simulink model "GS_model"  (R2018b)
settings: Solver=ode5  StartTime=0.0  StopTime=SimuStopTime  FixedStep=T_Simu  RelTol=1e-3
InitFcn:
  | Initial
undefined symbols (not defined in the file or in its folder): Aba10, Aba20, aeroCIP2006_S, aeroCIP2006_X, aeroCIP2006_Y, Agl0, Ass_kS, Ass_n1, Ass_n2, Ass_n3, Ass_n4, Ass_Noise, Ass_R, Ass_Resolution, Ass_TmOrder, AssA_Fix_Abs, AssB_Fix_Abs, AssC_Fix_Abs, AssD_Fix_Abs, AssE_Fix_Aps, AssF_Fix_Aps, C, c_max, c_min, Cd, CenterOfFigNX, CenterOfFigNY, CenterOfFigNZ, CenterOfFigP1, CenterOfFigP2, CenterOfFigPX, CenterOfFigPY, CenterOfFigPZ, Cmu, Crou, DEG2RAD, DiscIntNeverNeededParam, Eg_Dir, Eg_F, Eg_PrepareTime, Eg_r_L_L, Fw_Abf, Fw_Hmax, Fw_J, Fw_Spd0, Fw_Tmax, git_hash_BaseLine, git_hash_Project, Gnss_Noise_Pos, Gnss_Noise_Vel, Gnss_PropgationTime, GyroA_Fix_Abg, GyroA_Noise, GyroB_Fix_Abg, GyroB_Noise, GyroC_Fix_Abg, GyroC_Noise, GyroD_Fix_Abg, GyroD_Noise, h ... (+94)
libraries: simulink x308, sharedutil x46, aerolibutil x37, sharedtransform x31, vrlib x14, aerolibgravity2 x2
(part 18 of 20)

== system GS_model/Subsystem2/Subsystem/Sensor/Magnetometer/MmModel3/Mm_ErrSet/MmErrSet/MmErrSet_WildValue/MmAxisXErrSet_WildValue1 ==
  MmAxis_in : Inport
  ErrSwitch : Inport  Port=2
  MmAxis_Num : Inport  Port=3
  MmAxis_WildValue : Inport  Port=4
  Compare To Zero : simulink/Logic and Bit Operations/Compare To Zero  relop===  OutDataTypeStr=boolean
  Demux1 : Demux  Outputs=2
  Logical Operator : Logic  Operator=OR  AllPortsSameDT=off  OutDataTypeStr=boolean
  Relational Operator9 : RelationalOperator  Operator===  OutDataTypeStr=boolean  RndMeth=Simplest
  Switch1 : Switch  Criteria=u2 > Threshold  Threshold=0.5
  Triggered Subsystem8 : Subsystem  TreatAsAtomicUnit=on
  MmAxis_out : Outport
  wires:
  Logical Operator/1 -> Triggered Subsystem8/Enable
  Compare To Zero/1 -> Logical Operator/1
  Relational Operator9/1 -> Logical Operator/2
  Switch1/1 -> MmAxis_out/1
  MmAxis_in/1 -> Switch1/3
  Demux1/1 -> Relational Operator9/1, Compare To Zero/1
  Demux1/2 -> Triggered Subsystem8/1(In1)
  Triggered Subsystem8/1(Out1) -> Switch1/2
  MmAxis_Num/1 -> Relational Operator9/2
  MmAxis_WildValue/1 -> Switch1/1
  ErrSwitch/1 -> Demux1/1

== system GS_model/Subsystem2/Subsystem/Sensor/Magnetometer/MmModel3/Mm_ErrSet/MmErrSet/MmErrSet_WildValue/MmAxisXErrSet_WildValue2 ==
  MmAxis_in : Inport
  ErrSwitch : Inport  Port=2
  MmAxis_Num : Inport  Port=3
  MmAxis_WildValue : Inport  Port=4
  Compare To Zero : simulink/Logic and Bit Operations/Compare To Zero  relop===  OutDataTypeStr=boolean
  Demux1 : Demux  Outputs=2
  Logical Operator : Logic  Operator=OR  AllPortsSameDT=off  OutDataTypeStr=boolean
  Relational Operator9 : RelationalOperator  Operator===  OutDataTypeStr=boolean  RndMeth=Simplest
  Switch1 : Switch  Criteria=u2 > Threshold  Threshold=0.5
  Triggered Subsystem8 : Subsystem  TreatAsAtomicUnit=on
  MmAxis_out : Outport
  wires:
  ErrSwitch/1 -> Demux1/1
  MmAxis_WildValue/1 -> Switch1/1
  MmAxis_Num/1 -> Relational Operator9/2
  Triggered Subsystem8/1(Out1) -> Switch1/2
  Demux1/2 -> Triggered Subsystem8/1(In1)
  Demux1/1 -> Compare To Zero/1, Relational Operator9/1
  MmAxis_in/1 -> Switch1/3
  Switch1/1 -> MmAxis_out/1
  Relational Operator9/1 -> Logical Operator/2
  Compare To Zero/1 -> Logical Operator/1
  Logical Operator/1 -> Triggered Subsystem8/Enable

== system GS_model/Subsystem2/Subsystem/Sensor/Magnetometer/MmModel4/Mm_ErrSet/MmErrSet/MmErrSet_Constant/MmAxisXErrSet_Constant ==
  MmAxis_in : Inport
  ErrSwitch : Inport  Port=2
  MmAxis_Num : Inport  Port=3
  Compare To Zero : simulink/Logic and Bit Operations/Compare To Zero  relop===  OutDataTypeStr=boolean
  Demux1 : Demux  Outputs=2
  Logical Operator : Logic  Operator=OR  AllPortsSameDT=off  OutDataTypeStr=boolean
  Memory : Memory
  Relational Operator9 : RelationalOperator  Operator===  OutDataTypeStr=boolean  RndMeth=Simplest
  Switch1 : Switch  Criteria=u2 > Threshold  Threshold=0.5
  Triggered Subsystem8 : Subsystem  TreatAsAtomicUnit=on
  MmAxis_out : Outport
  wires:
  Logical Operator/1 -> Triggered Subsystem8/Enable
  Compare To Zero/1 -> Logical Operator/1
  Relational Operator9/1 -> Logical Operator/2
  MmAxis_Num/1 -> Relational Operator9/1
  Demux1/1 -> Relational Operator9/2, Compare To Zero/1
  Triggered Subsystem8/1(Out1) -> Switch1/2
  ErrSwitch/1 -> Demux1/1
  Memory/1 -> Switch1/1
  Demux1/2 -> Triggered Subsystem8/1(In1)
  MmAxis_in/1 -> Switch1/3
  Switch1/1 -> Memory/1, MmAxis_out/1

== system GS_model/Subsystem2/Subsystem/Sensor/Magnetometer/MmModel4/Mm_ErrSet/MmErrSet/MmErrSet_Constant/MmAxisXErrSet_Constant1 ==
  MmAxis_in : Inport
  ErrSwitch : Inport  Port=2
  MmAxis_Num : Inport  Port=3
  Compare To Zero : simulink/Logic and Bit Operations/Compare To Zero  relop===  OutDataTypeStr=boolean
  Demux1 : Demux  Outputs=2
  Logical Operator : Logic  Operator=OR  AllPortsSameDT=off  OutDataTypeStr=boolean
  Memory : Memory
  Relational Operator9 : RelationalOperator  Operator===  OutDataTypeStr=boolean  RndMeth=Simplest
  Switch1 : Switch  Criteria=u2 > Threshold  Threshold=0.5
  Triggered Subsystem8 : Subsystem  TreatAsAtomicUnit=on
  MmAxis_out : Outport
  wires:
  Switch1/1 -> MmAxis_out/1, Memory/1
  MmAxis_in/1 -> Switch1/3
  Demux1/2 -> Triggered Subsystem8/1(In1)
  Memory/1 -> Switch1/1
  ErrSwitch/1 -> Demux1/1
  Triggered Subsystem8/1(Out1) -> Switch1/2
  Demux1/1 -> Compare To Zero/1, Relational Operator9/2
  MmAxis_Num/1 -> Relational Operator9/1
  Relational Operator9/1 -> Logical Operator/2
  Compare To Zero/1 -> Logical Operator/1
  Logical Operator/1 -> Triggered Subsystem8/Enable

== system GS_model/Subsystem2/Subsystem/Sensor/Magnetometer/MmModel4/Mm_ErrSet/MmErrSet/MmErrSet_Constant/MmAxisXErrSet_Constant2 ==
  MmAxis_in : Inport
  ErrSwitch : Inport  Port=2
  MmAxis_Num : Inport  Port=3
  Compare To Zero : simulink/Logic and Bit Operations/Compare To Zero  relop===  OutDataTypeStr=boolean
  Demux1 : Demux  Outputs=2
  Logical Operator : Logic  Operator=OR  AllPortsSameDT=off  OutDataTypeStr=boolean
  Memory : Memory
  Relational Operator9 : RelationalOperator  Operator===  OutDataTypeStr=boolean  RndMeth=Simplest
  Switch1 : Switch  Criteria=u2 > Threshold  Threshold=0.5
  Triggered Subsystem8 : Subsystem  TreatAsAtomicUnit=on
  MmAxis_out : Outport
  wires:
  Logical Operator/1 -> Triggered Subsystem8/Enable
  Compare To Zero/1 -> Logical Operator/1
  Relational Operator9/1 -> Logical Operator/2
  MmAxis_Num/1 -> Relational Operator9/1
  Demux1/1 -> Relational Operator9/2, Compare To Zero/1
  Triggered Subsystem8/1(Out1) -> Switch1/2
  ErrSwitch/1 -> Demux1/1
  Memory/1 -> Switch1/1
  Demux1/2 -> Triggered Subsystem8/1(In1)
  MmAxis_in/1 -> Switch1/3
  Switch1/1 -> Memory/1, MmAxis_out/1

== system GS_model/Subsystem2/Subsystem/Sensor/Magnetometer/MmModel4/Mm_ErrSet/MmErrSet/MmErrSet_Jump/MmAxisXErrSet_Jump ==
  MmAxis_in : Inport
  ErrSet : Inport  Port=2
  MmAxis_Num : Inport  Port=3
  MmAxis_JumpSet : Inport  Port=4
  Add : Sum  Inputs=|++
  Compare To Zero : simulink/Logic and Bit Operations/Compare To Zero  relop===  OutDataTypeStr=boolean
  Demux1 : Demux
  Logical Operator : Logic  Operator=OR  AllPortsSameDT=off  OutDataTypeStr=boolean
  Product : Product
  Relational Operator9 : RelationalOperator  Operator===  OutDataTypeStr=boolean  RndMeth=Simplest
  Switch3 : Switch  Criteria=u2 > Threshold  Threshold=0.5
  Terminator : Terminator
  Triggered Subsystem8 : Subsystem  TreatAsAtomicUnit=on
  MmAxis_out : Outport
  wires:
  Logical Operator/1 -> Triggered Subsystem8/Enable
  Compare To Zero/1 -> Logical Operator/1
  Relational Operator9/1 -> Logical Operator/2
  Demux1/1 -> Relational Operator9/1, Compare To Zero/1  "Axis"
  Demux1/4 -> Product/2  "Coff"
  Triggered Subsystem8/1(Out1) -> Switch3/2
  Product/1 -> Add/1
  Demux1/2 -> Triggered Subsystem8/1(In1)  "Switch"
  MmAxis_in/1 -> Switch3/3, Add/2
  ErrSet/1 -> Demux1/1
  Add/1 -> Switch3/1
  Demux1/3 -> Terminator/1  "Period"
  MmAxis_Num/1 -> Relational Operator9/2
  Switch3/1 -> MmAxis_out/1
  MmAxis_JumpSet/1 -> Product/1

== system GS_model/Subsystem2/Subsystem/Sensor/Magnetometer/MmModel4/Mm_ErrSet/MmErrSet/MmErrSet_Jump/MmAxisXErrSet_Jump1 ==
  MmAxis_in : Inport
  ErrSet : Inport  Port=2
  MmAxis_Num : Inport  Port=3
  MmAxis_JumpSet : Inport  Port=4
  Add : Sum  Inputs=|++
  Compare To Zero : simulink/Logic and Bit Operations/Compare To Zero  relop===  OutDataTypeStr=boolean
  Demux1 : Demux
  Logical Operator : Logic  Operator=OR  AllPortsSameDT=off  OutDataTypeStr=boolean
  Product : Product
  Relational Operator9 : RelationalOperator  Operator===  OutDataTypeStr=boolean  RndMeth=Simplest
  Switch3 : Switch  Criteria=u2 > Threshold  Threshold=0.5
  Terminator : Terminator
  Triggered Subsystem8 : Subsystem  TreatAsAtomicUnit=on
  MmAxis_out : Outport
  wires:
  MmAxis_JumpSet/1 -> Product/1
  Switch3/1 -> MmAxis_out/1
  MmAxis_Num/1 -> Relational Operator9/2
  Demux1/3 -> Terminator/1  "Period"
  Add/1 -> Switch3/1
  ErrSet/1 -> Demux1/1
  MmAxis_in/1 -> Add/2, Switch3/3
  Demux1/2 -> Triggered Subsystem8/1(In1)  "Switch"
  Product/1 -> Add/1
  Triggered Subsystem8/1(Out1) -> Switch3/2
  Demux1/4 -> Product/2  "Coff"
  Demux1/1 -> Compare To Zero/1, Relational Operator9/1  "Axis"
  Relational Operator9/1 -> Logical Operator/2
  Compare To Zero/1 -> Logical Operator/1
  Logical Operator/1 -> Triggered Subsystem8/Enable

== system GS_model/Subsystem2/Subsystem/Sensor/Magnetometer/MmModel4/Mm_ErrSet/MmErrSet/MmErrSet_Jump/MmAxisXErrSet_Jump2 ==
  MmAxis_in : Inport
  ErrSet : Inport  Port=2
  MmAxis_Num : Inport  Port=3
  MmAxis_JumpSet : Inport  Port=4
  Add : Sum  Inputs=|++
  Compare To Zero : simulink/Logic and Bit Operations/Compare To Zero  relop===  OutDataTypeStr=boolean
  Demux1 : Demux
  Logical Operator : Logic  Operator=OR  AllPortsSameDT=off  OutDataTypeStr=boolean
  Product : Product
  Relational Operator9 : RelationalOperator  Operator===  OutDataTypeStr=boolean  RndMeth=Simplest
  Switch3 : Switch  Criteria=u2 > Threshold  Threshold=0.5
  Terminator : Terminator
  Triggered Subsystem8 : Subsystem  TreatAsAtomicUnit=on
  MmAxis_out : Outport
  wires:
  Logical Operator/1 -> Triggered Subsystem8/Enable
  Compare To Zero/1 -> Logical Operator/1
  Relational Operator9/1 -> Logical Operator/2
  Demux1/1 -> Relational Operator9/1, Compare To Zero/1  "Axis"
  Demux1/4 -> Product/2  "Coff"
  Triggered Subsystem8/1(Out1) -> Switch3/2
  Product/1 -> Add/1
  Demux1/2 -> Triggered Subsystem8/1(In1)  "Switch"
  MmAxis_in/1 -> Switch3/3, Add/2
  ErrSet/1 -> Demux1/1
  Add/1 -> Switch3/1
  Demux1/3 -> Terminator/1  "Period"
  MmAxis_Num/1 -> Relational Operator9/2
  Switch3/1 -> MmAxis_out/1
  MmAxis_JumpSet/1 -> Product/1

== system GS_model/Subsystem2/Subsystem/Sensor/Magnetometer/MmModel4/Mm_ErrSet/MmErrSet/MmErrSet_Wave/MmAxisXErrSet_Wave ==
  MmAxis_in : Inport
  ErrSet : Inport  Port=2
  MmAxis_Num : Inport  Port=3
  MmAxis_WaveSet : Inport  Port=4
  Add : Sum  Inputs=|++
  Compare To Zero : simulink/Logic and Bit Operations/Compare To Zero  relop===  OutDataTypeStr=boolean
  Demux1 : Demux  Outputs=3
  Logical Operator : Logic  Operator=OR  AllPortsSameDT=off  OutDataTypeStr=boolean
  Product : Product
  Relational Operator9 : RelationalOperator  Operator===  OutDataTypeStr=boolean  RndMeth=Simplest
  Switch3 : Switch  Criteria=u2 > Threshold  Threshold=0.5
  Triggered Subsystem8 : Subsystem  TreatAsAtomicUnit=on
  MmAxis_out : Outport
  wires:
  Compare To Zero/1 -> Logical Operator/1
  Logical Operator/1 -> Triggered Subsystem8/Enable
  Relational Operator9/1 -> Logical Operator/2
  MmAxis_WaveSet/1 -> Product/1
  Product/1 -> Add/1
  ErrSet/1 -> Demux1/1
  Add/1 -> Switch3/1
  MmAxis_in/1 -> Add/2, Switch3/3
  Demux1/2 -> Triggered Subsystem8/1(In1)  "Switch"
  Demux1/1 -> Relational Operator9/1, Compare To Zero/1  "Axis"
  Demux1/3 -> Product/2  "Coff"
  MmAxis_Num/1 -> Relational Operator9/2
  Switch3/1 -> MmAxis_out/1
  Triggered Subsystem8/1(Out1) -> Switch3/2

== system GS_model/Subsystem2/Subsystem/Sensor/Magnetometer/MmModel4/Mm_ErrSet/MmErrSet/MmErrSet_Wave/MmAxisXErrSet_Wave1 ==
  MmAxis_in : Inport
  ErrSet : Inport  Port=2
  MmAxis_Num : Inport  Port=3
  MmAxis_WaveSet : Inport  Port=4
  Add : Sum  Inputs=|++
  Compare To Zero : simulink/Logic and Bit Operations/Compare To Zero  relop===  OutDataTypeStr=boolean
  Demux1 : Demux  Outputs=3
  Logical Operator : Logic  Operator=OR  AllPortsSameDT=off  OutDataTypeStr=boolean
  Product : Product
  Relational Operator9 : RelationalOperator  Operator===  OutDataTypeStr=boolean  RndMeth=Simplest
  Switch3 : Switch  Criteria=u2 > Threshold  Threshold=0.5
  Triggered Subsystem8 : Subsystem  TreatAsAtomicUnit=on
  MmAxis_out : Outport
  wires:
  Triggered Subsystem8/1(Out1) -> Switch3/2
  Switch3/1 -> MmAxis_out/1
  MmAxis_Num/1 -> Relational Operator9/2
  Demux1/3 -> Product/2  "Coff"
  Demux1/1 -> Compare To Zero/1, Relational Operator9/1  "Axis"
  Demux1/2 -> Triggered Subsystem8/1(In1)  "Switch"
  MmAxis_in/1 -> Switch3/3, Add/2
  Add/1 -> Switch3/1
  ErrSet/1 -> Demux1/1
  Product/1 -> Add/1
  MmAxis_WaveSet/1 -> Product/1
  Relational Operator9/1 -> Logical Operator/2
  Logical Operator/1 -> Triggered Subsystem8/Enable
  Compare To Zero/1 -> Logical Operator/1

== system GS_model/Subsystem2/Subsystem/Sensor/Magnetometer/MmModel4/Mm_ErrSet/MmErrSet/MmErrSet_Wave/MmAxisXErrSet_Wave2 ==
  MmAxis_in : Inport
  ErrSet : Inport  Port=2
  MmAxis_Num : Inport  Port=3
  MmAxis_WaveSet : Inport  Port=4
  Add : Sum  Inputs=|++
  Compare To Zero : simulink/Logic and Bit Operations/Compare To Zero  relop===  OutDataTypeStr=boolean
  Demux1 : Demux  Outputs=3
  Logical Operator : Logic  Operator=OR  AllPortsSameDT=off  OutDataTypeStr=boolean
  Product : Product
  Relational Operator9 : RelationalOperator  Operator===  OutDataTypeStr=boolean  RndMeth=Simplest
  Switch3 : Switch  Criteria=u2 > Threshold  Threshold=0.5
  Triggered Subsystem8 : Subsystem  TreatAsAtomicUnit=on
  MmAxis_out : Outport
  wires:
  Compare To Zero/1 -> Logical Operator/1
  Logical Operator/1 -> Triggered Subsystem8/Enable
  Relational Operator9/1 -> Logical Operator/2
  MmAxis_WaveSet/1 -> Product/1
  Product/1 -> Add/1
  ErrSet/1 -> Demux1/1
  Add/1 -> Switch3/1
  MmAxis_in/1 -> Add/2, Switch3/3
  Demux1/2 -> Triggered Subsystem8/1(In1)  "Switch"
  Demux1/1 -> Relational Operator9/1, Compare To Zero/1  "Axis"
  Demux1/3 -> Product/2  "Coff"
  MmAxis_Num/1 -> Relational Operator9/2
  Switch3/1 -> MmAxis_out/1
  Triggered Subsystem8/1(Out1) -> Switch3/2

== system GS_model/Subsystem2/Subsystem/Sensor/Magnetometer/MmModel4/Mm_ErrSet/MmErrSet/MmErrSet_WildValue/MmAxisXErrSet_WildValue ==
  MmAxis_in : Inport
  ErrSwitch : Inport  Port=2
  MmAxis_Num : Inport  Port=3
  MmAxis_WildValue : Inport  Port=4
  Compare To Zero : simulink/Logic and Bit Operations/Compare To Zero  relop===  OutDataTypeStr=boolean
  Demux1 : Demux  Outputs=2
  Logical Operator : Logic  Operator=OR  AllPortsSameDT=off  OutDataTypeStr=boolean
  Relational Operator9 : RelationalOperator  Operator===  OutDataTypeStr=boolean  RndMeth=Simplest
  Switch1 : Switch  Criteria=u2 > Threshold  Threshold=0.5
  Triggered Subsystem8 : Subsystem  TreatAsAtomicUnit=on
  MmAxis_out : Outport
  wires:
  Logical Operator/1 -> Triggered Subsystem8/Enable
  Compare To Zero/1 -> Logical Operator/1
  Relational Operator9/1 -> Logical Operator/2
  Switch1/1 -> MmAxis_out/1
  MmAxis_in/1 -> Switch1/3
  Demux1/1 -> Relational Operator9/1, Compare To Zero/1
  Demux1/2 -> Triggered Subsystem8/1(In1)
  Triggered Subsystem8/1(Out1) -> Switch1/2
  MmAxis_Num/1 -> Relational Operator9/2
  MmAxis_WildValue/1 -> Switch1/1
  ErrSwitch/1 -> Demux1/1

== system GS_model/Subsystem2/Subsystem/Sensor/Magnetometer/MmModel4/Mm_ErrSet/MmErrSet/MmErrSet_WildValue/MmAxisXErrSet_WildValue1 ==
  MmAxis_in : Inport
  ErrSwitch : Inport  Port=2
  MmAxis_Num : Inport  Port=3
  MmAxis_WildValue : Inport  Port=4
  Compare To Zero : simulink/Logic and Bit Operations/Compare To Zero  relop===  OutDataTypeStr=boolean
  Demux1 : Demux  Outputs=2
  Logical Operator : Logic  Operator=OR  AllPortsSameDT=off  OutDataTypeStr=boolean
  Relational Operator9 : RelationalOperator  Operator===  OutDataTypeStr=boolean  RndMeth=Simplest
  Switch1 : Switch  Criteria=u2 > Threshold  Threshold=0.5
  Triggered Subsystem8 : Subsystem  TreatAsAtomicUnit=on
  MmAxis_out : Outport
  wires:
  ErrSwitch/1 -> Demux1/1
  MmAxis_WildValue/1 -> Switch1/1
  MmAxis_Num/1 -> Relational Operator9/2
  Triggered Subsystem8/1(Out1) -> Switch1/2
  Demux1/2 -> Triggered Subsystem8/1(In1)
  Demux1/1 -> Compare To Zero/1, Relational Operator9/1
  MmAxis_in/1 -> Switch1/3
  Switch1/1 -> MmAxis_out/1
  Relational Operator9/1 -> Logical Operator/2
  Compare To Zero/1 -> Logical Operator/1
  Logical Operator/1 -> Triggered Subsystem8/Enable

== system GS_model/Subsystem2/Subsystem/Sensor/Magnetometer/MmModel4/Mm_ErrSet/MmErrSet/MmErrSet_WildValue/MmAxisXErrSet_WildValue2 ==
  MmAxis_in : Inport
  ErrSwitch : Inport  Port=2
  MmAxis_Num : Inport  Port=3
  MmAxis_WildValue : Inport  Port=4
  Compare To Zero : simulink/Logic and Bit Operations/Compare To Zero  relop===  OutDataTypeStr=boolean
  Demux1 : Demux  Outputs=2
  Logical Operator : Logic  Operator=OR  AllPortsSameDT=off  OutDataTypeStr=boolean
  Relational Operator9 : RelationalOperator  Operator===  OutDataTypeStr=boolean  RndMeth=Simplest
  Switch1 : Switch  Criteria=u2 > Threshold  Threshold=0.5
  Triggered Subsystem8 : Subsystem  TreatAsAtomicUnit=on
  MmAxis_out : Outport
  wires:
  Logical Operator/1 -> Triggered Subsystem8/Enable
  Compare To Zero/1 -> Logical Operator/1
  Relational Operator9/1 -> Logical Operator/2
  Switch1/1 -> MmAxis_out/1
  MmAxis_in/1 -> Switch1/3
  Demux1/1 -> Relational Operator9/1, Compare To Zero/1
  Demux1/2 -> Triggered Subsystem8/1(In1)
  Triggered Subsystem8/1(Out1) -> Switch1/2
  MmAxis_Num/1 -> Relational Operator9/2
  MmAxis_WildValue/1 -> Switch1/1
  ErrSwitch/1 -> Demux1/1

== system GS_model/Subsystem2/Subsystem/PhysicsModel/Environment/Sun  press torque/Sun  press torque2/Sun  press torque/+Y SunPanel/Compute press of sun radiation/1//r ==
  In1 : Inport
  If : If  IfExpression=u1== 0
  If Action Subsystem1 : Subsystem  TreatAsAtomicUnit=on
  If Action Subsystem2 : Subsystem  TreatAsAtomicUnit=on
  Merge : Merge
  Out1 : Outport
  wires:
  In1/1 -> If Action Subsystem1/1(In1), If/1
  Merge/1 -> Out1/1
  If Action Subsystem2/1(Out1) -> Merge/1
  If Action Subsystem1/1(Out1) -> Merge/2
  If/2 -> If Action Subsystem1/Action
  If/1 -> If Action Subsystem2/Action

== system GS_model/Subsystem2/Subsystem/PhysicsModel/Environment/Sun  press torque/Sun  press torque2/Sun  press torque/-Y SunPanel/Compute press of sun radiation/1//r ==
  In1 : Inport
  If : If  IfExpression=u1== 0
  If Action Subsystem1 : Subsystem  TreatAsAtomicUnit=on
  If Action Subsystem2 : Subsystem  TreatAsAtomicUnit=on
  Merge : Merge
  Out1 : Outport
  wires:
  If/1 -> If Action Subsystem2/Action
  If/2 -> If Action Subsystem1/Action
  If Action Subsystem1/1(Out1) -> Merge/2
  If Action Subsystem2/1(Out1) -> Merge/1
  Merge/1 -> Out1/1
  In1/1 -> If/1, If Action Subsystem1/1(In1)

== system GS_model/Subsystem2/Subsystem/PhysicsModel/Environment/Sun  press torque/Sun  press torque2/Sun  press torque/Torque from   satalite board/Torque from  board perpendicular to z axis /Compute press of sun radiation ==
  note: u_n
  note: u_t
  Sun Orientation : Inport
  TC_SunPressCoeff : Inport  Port=2
  1/r : Subsystem  TreatAsAtomicUnit=on
  3x3 Cross Product : sharedutil/3x3 Cross Product  aMode=aMode
      settings: SourceProductBaseCode=AE,PW,MT,VE,VP
  3x3 Cross Product1 : sharedutil/3x3 Cross Product  aMode=aMode
      settings: SourceProductBaseCode=AE,PW,MT,VE,VP
  Board Orientation : Constant  Value=n_NZ  VectorParams1D=off
  Board Orientation1 : Constant  Value=n_PZ  VectorParams1D=off
  Board Orientation2 : Constant  Value=Szp_board  VectorParams1D=off
  Board Orientation3 : Constant  Value=Szn_board  VectorParams1D=off
  Crd2 : Constant  Value=2/3*Crou*Cmu
  Dot Product : DotProduct  InputSameDT=on  OutDataTypeStr=Inherit: Inherit via internal rule
  Dot Product1 : DotProduct  InputSameDT=on  OutDataTypeStr=Inherit: Inherit via internal rule
  Fcn : Fcn  Expr=u(3)
  Fcn1 : Fcn  Expr=u(3)
  Gain : Gain  Gain=1+Crou*(1-Cmu)
  Gain1 : Gain  Gain=-1  SaturateOnIntegerOverflow=on  OutDataTypeStr=Inherit: Same as input  ParamDataTypeStr=Inherit: Same as input
  Gain2 : Gain  Gain=SConst/C
  Gain3 : Gain  Gain=1-Crou+Crou*Cmu
  Product{1..6} (6 alike) : Product  SaturateOnIntegerOverflow=on  OutDataTypeStr=Inherit: Same as first input
  Sum1 : Sum  SaturateOnIntegerOverflow=on  InputSameDT=on  OutDataTypeStr=Inherit: Same as first input
  Sum2 : Sum  Inputs=|++  SaturateOnIntegerOverflow=on  InputSameDT=on  OutDataTypeStr=Inherit: Same as first input
  Switch1 : Switch  SaturateOnIntegerOverflow=on  InputSameDT=on
  Switch2 : Switch  SaturateOnIntegerOverflow=on  InputSameDT=on
  Trigonometric Function1 : Trigonometry
  Trigonometric Function2 : Trigonometry  Operator=acos
  Fz : Outport
  wires:
  Board Orientation1/1 -> Switch2/1
  Board Orientation/1 -> Switch2/3
  Fcn/1 -> Switch2/2
  Gain/1 -> Sum2/1
  Sum2/1 -> Product4/1
  Crd2/1 -> Sum2/2
  Gain1/1 -> Product4/2
  Switch2/1 -> Dot Product/2, Gain1/1, 3x3 Cross Product1/2, 3x3 Cross Product/2
  Sum1/1 -> Product3/1
  Sun Orientation/1 -> Fcn1/1, Fcn/1, 3x3 Cross Product/1, Dot Product/1
  Trigonometric Function2/1 -> Trigonometric Function1/1
  Gain3/1 -> Product2/2
  3x3 Cross Product/1 -> 3x3 Cross Product1/1
  1/r/1(Out1) -> Product1/2
  3x3 Cross Product1/1 -> Dot Product1/1, Product1/1, Dot Product1/2
  Product2/1 -> Sum1/1
  Product4/1 -> Sum1/2
  Product1/1 -> Product2/1
  Trigonometric Function1/1 -> Gain3/1
  Dot Product1/1 -> 1/r/1(In1)
  Product3/1 -> Fz/1
  Board Orientation2/1 -> Switch1/1
  Board Orientation3/1 -> Switch1/3
  Fcn1/1 -> Switch1/2
  Dot Product/1 -> Product5/2, Gain/1, Trigonometric Function2/1
  Product5/1 -> Gain2/1
  Switch1/1 -> Product5/1
  Gain2/1 -> Product6/1
  TC_SunPressCoeff/1 -> Product6/2
  Product6/1 -> Product3/2

== system GS_model/Subsystem2/Subsystem/PhysicsModel/Environment/Sun  press torque/Sun  press torque2/Sun  press torque/Torque from   satalite board/Torque from  board perpendicular to z axis /compute centroi 1 ==
  Orientation : Inport
  Cent : Inport  Port=2
  Fcn : Fcn  Expr=u(3)
  Sum2 : Sum  Inputs=|+-
  Switch1 : Switch  SaturateOnIntegerOverflow=on  InputSameDT=on
  y2 : Constant  Value=CenterOfFigNZ  VectorParams1D=off
  y3 : Constant  Value=CenterOfFigPZ  VectorParams1D=off
  r_z : Outport
  wires:
  Sum2/1 -> r_z/1
  y3/1 -> Switch1/1
  y2/1 -> Switch1/3
  Fcn/1 -> Switch1/2
  Orientation/1 -> Fcn/1
  Cent/1 -> Sum2/2
  Switch1/1 -> Sum2/1

== system GS_model/Subsystem2/Subsystem/PhysicsModel/Environment/Sun  press torque/Sun  press torque2/Sun  press torque/Torque from   satalite board/Torque from board perpendicular to x axis/Compute press of sun radiation ==
  note: cos_theta
  note: u_n
  note: u_t
  note: Huang zhen gui P67
  Sun Orientation : Inport
  TC_SunPressCoeff : Inport  Port=2
  1/r : Subsystem  TreatAsAtomicUnit=on
  3x3 Cross Product : sharedutil/3x3 Cross Product  aMode=aMode
      settings: SourceProductBaseCode=AE,PW,MT,VE,VP
  3x3 Cross Product1 : sharedutil/3x3 Cross Product  aMode=aMode
      settings: SourceProductBaseCode=AE,PW,MT,VE,VP
  Board Orientation : Constant  Value=n_NX  VectorParams1D=off
  Board Orientation1 : Constant  Value=n_PX  VectorParams1D=off
  Crd2 : Constant  Value=2/3*Crou*Cmu
  Dot Product : DotProduct  InputSameDT=on  OutDataTypeStr=Inherit: Inherit via internal rule
  Dot Product1 : DotProduct  InputSameDT=on  OutDataTypeStr=Inherit: Inherit via internal rule
  Fcn : Fcn  Expr=u(1)
  Gain : Gain  Gain=1+Crou*(1-Cmu)
  Gain1 : Gain  Gain=-1  SaturateOnIntegerOverflow=on  OutDataTypeStr=Inherit: Same as input  ParamDataTypeStr=Inherit: Same as input
  Gain2 : Gain  Gain=SConst/C*Sx_board
  Gain4 : Gain  Gain=1-Crou+Crou*Cmu
  Product : Product
  Product{1..4} (4 alike) : Product  SaturateOnIntegerOverflow=on  OutDataTypeStr=Inherit: Same as first input
  Sum1 : Sum  SaturateOnIntegerOverflow=on  InputSameDT=on  OutDataTypeStr=Inherit: Same as first input
  Sum2 : Sum  Inputs=|++  SaturateOnIntegerOverflow=on  InputSameDT=on  OutDataTypeStr=Inherit: Same as first input
  Switch2 : Switch  SaturateOnIntegerOverflow=on  InputSameDT=on
  Trigonometric Function1 : Trigonometry
  Trigonometric Function2 : Trigonometry  Operator=acos
  Fx : Outport
  wires:
  Board Orientation1/1 -> Switch2/1
  Board Orientation/1 -> Switch2/3
  Fcn/1 -> Switch2/2
  Gain/1 -> Sum2/1
  Sum2/1 -> Product4/1
  Crd2/1 -> Sum2/2
  Gain1/1 -> Product4/2
  Switch2/1 -> Gain1/1, 3x3 Cross Product1/2, 3x3 Cross Product/2, Dot Product/1
  Sum1/1 -> Product3/1
  Dot Product/1 -> Gain2/1, Gain/1, Trigonometric Function2/1
  Sun Orientation/1 -> Fcn/1, Dot Product/2, 3x3 Cross Product/1
  Trigonometric Function2/1 -> Trigonometric Function1/1
  Gain4/1 -> Product2/2
  3x3 Cross Product/1 -> 3x3 Cross Product1/1
  1/r/1(Out1) -> Product1/2
  3x3 Cross Product1/1 -> Dot Product1/2, Dot Product1/1, Product1/1
  Product3/1 -> Fx/1
  Product2/1 -> Sum1/1
  Product4/1 -> Sum1/2
  Product1/1 -> Product2/1
  Trigonometric Function1/1 -> Gain4/1
  Dot Product1/1 -> 1/r/1(In1)
  Gain2/1 -> Product/1
  TC_SunPressCoeff/1 -> Product/2
  Product/1 -> Product3/2

== system GS_model/Subsystem2/Subsystem/PhysicsModel/Environment/Sun  press torque/Sun  press torque2/Sun  press torque/Torque from   satalite board/Torque from board perpendicular to x axis/compute centroi 1 ==
  Orientation : Inport
  Cent : Inport  Port=2
  Fcn : Fcn  Expr=u(1)
  Sum2 : Sum  Inputs=|+-
  Switch1 : Switch  SaturateOnIntegerOverflow=on  InputSameDT=on
  y2 : Constant  Value=CenterOfFigNX  VectorParams1D=off
  y3 : Constant  Value=CenterOfFigPX  VectorParams1D=off
  r_x : Outport
  wires:
  Sum2/1 -> r_x/1
  y3/1 -> Switch1/1
  y2/1 -> Switch1/3
  Fcn/1 -> Switch1/2
  Orientation/1 -> Fcn/1
  Cent/1 -> Sum2/2
  Switch1/1 -> Sum2/1

== system GS_model/Subsystem2/Subsystem/PhysicsModel/Environment/Sun  press torque/Sun  press torque2/Sun  press torque/Torque from   satalite board/Torque from board perpendicular to y axis/Compute press of sun radiation1 ==
  note: cos_theta
  note: u_n
  note: u_t
  note: Huang zhen gui P67
  Sun Orientation : Inport
  TC_SunPressCoeff : Inport  Port=2
  1/r : Subsystem  TreatAsAtomicUnit=on
  3x3 Cross Product : sharedutil/3x3 Cross Product  aMode=aMode
      settings: SourceProductBaseCode=AE,PW,MT,VE,VP
  3x3 Cross Product1 : sharedutil/3x3 Cross Product  aMode=aMode
      settings: SourceProductBaseCode=AE,PW,MT,VE,VP
  Board Orientation : Constant  Value=n_NY  VectorParams1D=off
  Board Orientation1 : Constant  Value=n_PY  VectorParams1D=off
  Crd2 : Constant  Value=2/3*Crou*Cmu
  Dot Product : DotProduct  InputSameDT=on  OutDataTypeStr=Inherit: Inherit via internal rule
  Dot Product1 : DotProduct  InputSameDT=on  OutDataTypeStr=Inherit: Inherit via internal rule
  Fcn : Fcn  Expr=u(2)
  Gain : Gain  Gain=1+Crou*(1-Cmu)
  Gain1 : Gain  Gain=-1  SaturateOnIntegerOverflow=on  OutDataTypeStr=Inherit: Same as input  ParamDataTypeStr=Inherit: Same as input
  Gain2 : Gain  Gain=SConst/C*Sy_board
  Gain4 : Gain  Gain=1-Crou+Crou*Cmu
  Product : Product
  Product{1..4} (4 alike) : Product  SaturateOnIntegerOverflow=on  OutDataTypeStr=Inherit: Same as first input
  Sum1 : Sum  SaturateOnIntegerOverflow=on  InputSameDT=on  OutDataTypeStr=Inherit: Same as first input
  Sum2 : Sum  Inputs=|++  SaturateOnIntegerOverflow=on  InputSameDT=on  OutDataTypeStr=Inherit: Same as first input
  Switch2 : Switch  SaturateOnIntegerOverflow=on  InputSameDT=on
  Trigonometric Function1 : Trigonometry
  Trigonometric Function2 : Trigonometry  Operator=acos
  Fy : Outport
  wires:
  Board Orientation1/1 -> Switch2/1
  Board Orientation/1 -> Switch2/3
  Fcn/1 -> Switch2/2
  Gain/1 -> Sum2/1
  Sum2/1 -> Product4/1
  Crd2/1 -> Sum2/2
  Gain1/1 -> Product4/2
  Switch2/1 -> Gain1/1, 3x3 Cross Product1/2, 3x3 Cross Product/2, Dot Product/1
  Sum1/1 -> Product3/1
  Dot Product/1 -> Gain2/1, Gain/1, Trigonometric Function2/1
  Sun Orientation/1 -> Fcn/1, Dot Product/2, 3x3 Cross Product/1
  Trigonometric Function2/1 -> Trigonometric Function1/1
  Gain4/1 -> Product2/2
  3x3 Cross Product/1 -> 3x3 Cross Product1/1
  1/r/1(Out1) -> Product1/2
  3x3 Cross Product1/1 -> Dot Product1/2, Dot Product1/1, Product1/1
  Product3/1 -> Fy/1
  Product2/1 -> Sum1/1
  Product4/1 -> Sum1/2
  Product1/1 -> Product2/1
  Trigonometric Function1/1 -> Gain4/1
  Dot Product1/1 -> 1/r/1(In1)
  Gain2/1 -> Product/1
  TC_SunPressCoeff/1 -> Product/2
  Product/1 -> Product3/2

== system GS_model/Subsystem2/Subsystem/PhysicsModel/Environment/Sun  press torque/Sun  press torque2/Sun  press torque/Torque from   satalite board/Torque from board perpendicular to y axis/compute centroi 1 ==
  Orientation : Inport
  Cent : Inport  Port=2
  Fcn : Fcn  Expr=u(2)
  Sum2 : Sum  Inputs=|+-
  Switch1 : Switch  SaturateOnIntegerOverflow=on  InputSameDT=on
  y2 : Constant  Value=CenterOfFigNY  VectorParams1D=off
  y3 : Constant  Value=CenterOfFigPY  VectorParams1D=off
  r_y : Outport
  wires:
  Sum2/1 -> r_y/1
  y3/1 -> Switch1/1
  y2/1 -> Switch1/3
  Fcn/1 -> Switch1/2
  Orientation/1 -> Fcn/1
  Cent/1 -> Sum2/2
  Switch1/1 -> Sum2/1

== system GS_model/Subsystem2/Subsystem/Sensor/Magnetometer/MmModel1/Mm_ErrSet/MmErrSet/MmErrSet_Constant/MmAxisXErrSet_Constant/Triggered Subsystem8 ==
  In1 : Inport
  Enable : EnablePort
  Out1 : Outport
  wires:
  In1/1 -> Out1/1

== system GS_model/Subsystem2/Subsystem/Sensor/Magnetometer/MmModel1/Mm_ErrSet/MmErrSet/MmErrSet_Constant/MmAxisXErrSet_Constant1/Triggered Subsystem8 ==
  In1 : Inport
  Enable : EnablePort
  Out1 : Outport
  wires:
  In1/1 -> Out1/1

== system GS_model/Subsystem2/Subsystem/Sensor/Magnetometer/MmModel1/Mm_ErrSet/MmErrSet/MmErrSet_Constant/MmAxisXErrSet_Constant2/Triggered Subsystem8 ==
  In1 : Inport
  Enable : EnablePort
  Out1 : Outport
  wires:
  In1/1 -> Out1/1

== system GS_model/Subsystem2/Subsystem/Sensor/Magnetometer/MmModel1/Mm_ErrSet/MmErrSet/MmErrSet_Jump/MmAxisXErrSet_Jump/Triggered Subsystem8 ==
  In1 : Inport
  Enable : EnablePort
  Out1 : Outport
  wires:
  In1/1 -> Out1/1

== system GS_model/Subsystem2/Subsystem/Sensor/Magnetometer/MmModel1/Mm_ErrSet/MmErrSet/MmErrSet_Jump/MmAxisXErrSet_Jump1/Triggered Subsystem8 ==
  In1 : Inport
  Enable : EnablePort
  Out1 : Outport
  wires:
  In1/1 -> Out1/1

== system GS_model/Subsystem2/Subsystem/Sensor/Magnetometer/MmModel1/Mm_ErrSet/MmErrSet/MmErrSet_Jump/MmAxisXErrSet_Jump2/Triggered Subsystem8 ==
  In1 : Inport
  Enable : EnablePort
  Out1 : Outport
  wires:
  In1/1 -> Out1/1

== system GS_model/Subsystem2/Subsystem/Sensor/Magnetometer/MmModel1/Mm_ErrSet/MmErrSet/MmErrSet_Wave/MmAxisXErrSet_Wave/Triggered Subsystem8 ==
  In1 : Inport
  Enable : EnablePort
  Out1 : Outport
  wires:
  In1/1 -> Out1/1

== system GS_model/Subsystem2/Subsystem/Sensor/Magnetometer/MmModel1/Mm_ErrSet/MmErrSet/MmErrSet_Wave/MmAxisXErrSet_Wave1/Triggered Subsystem8 ==
  In1 : Inport
  Enable : EnablePort
  Out1 : Outport
  wires:
  In1/1 -> Out1/1

== system GS_model/Subsystem2/Subsystem/Sensor/Magnetometer/MmModel1/Mm_ErrSet/MmErrSet/MmErrSet_Wave/MmAxisXErrSet_Wave2/Triggered Subsystem8 ==
  In1 : Inport
  Enable : EnablePort
  Out1 : Outport
  wires:
  In1/1 -> Out1/1

== system GS_model/Subsystem2/Subsystem/Sensor/Magnetometer/MmModel1/Mm_ErrSet/MmErrSet/MmErrSet_WildValue/MmAxisXErrSet_WildValue/Triggered Subsystem8 ==
  In1 : Inport
  Enable : EnablePort
  Out1 : Outport
  wires:
  In1/1 -> Out1/1

== system GS_model/Subsystem2/Subsystem/Sensor/Magnetometer/MmModel1/Mm_ErrSet/MmErrSet/MmErrSet_WildValue/MmAxisXErrSet_WildValue1/Triggered Subsystem8 ==
  In1 : Inport
  Enable : EnablePort
  Out1 : Outport
  wires:
  In1/1 -> Out1/1

== system GS_model/Subsystem2/Subsystem/Sensor/Magnetometer/MmModel1/Mm_ErrSet/MmErrSet/MmErrSet_WildValue/MmAxisXErrSet_WildValue2/Triggered Subsystem8 ==
  In1 : Inport
  Enable : EnablePort
  Out1 : Outport
  wires:
  In1/1 -> Out1/1

== system GS_model/Subsystem2/Subsystem/Sensor/Magnetometer/MmModel2/Mm_ErrSet/MmErrSet/MmErrSet_Constant/MmAxisXErrSet_Constant/Triggered Subsystem8 ==
  In1 : Inport
  Enable : EnablePort
  Out1 : Outport
  wires:
  In1/1 -> Out1/1

== system GS_model/Subsystem2/Subsystem/Sensor/Magnetometer/MmModel2/Mm_ErrSet/MmErrSet/MmErrSet_Constant/MmAxisXErrSet_Constant1/Triggered Subsystem8 ==
  In1 : Inport
  Enable : EnablePort
  Out1 : Outport
  wires:
  In1/1 -> Out1/1

== system GS_model/Subsystem2/Subsystem/Sensor/Magnetometer/MmModel2/Mm_ErrSet/MmErrSet/MmErrSet_Constant/MmAxisXErrSet_Constant2/Triggered Subsystem8 ==
  In1 : Inport
  Enable : EnablePort
  Out1 : Outport
  wires:
  In1/1 -> Out1/1

== system GS_model/Subsystem2/Subsystem/Sensor/Magnetometer/MmModel2/Mm_ErrSet/MmErrSet/MmErrSet_Jump/MmAxisXErrSet_Jump/Triggered Subsystem8 ==
  In1 : Inport
  Enable : EnablePort
  Out1 : Outport
  wires:
  In1/1 -> Out1/1

== system GS_model/Subsystem2/Subsystem/Sensor/Magnetometer/MmModel2/Mm_ErrSet/MmErrSet/MmErrSet_Jump/MmAxisXErrSet_Jump1/Triggered Subsystem8 ==
  In1 : Inport
  Enable : EnablePort
  Out1 : Outport
  wires:
  In1/1 -> Out1/1

== system GS_model/Subsystem2/Subsystem/Sensor/Magnetometer/MmModel2/Mm_ErrSet/MmErrSet/MmErrSet_Jump/MmAxisXErrSet_Jump2/Triggered Subsystem8 ==
  In1 : Inport
  Enable : EnablePort
  Out1 : Outport
  wires:
  In1/1 -> Out1/1

== system GS_model/Subsystem2/Subsystem/Sensor/Magnetometer/MmModel2/Mm_ErrSet/MmErrSet/MmErrSet_Wave/MmAxisXErrSet_Wave/Triggered Subsystem8 ==
  In1 : Inport
  Enable : EnablePort
  Out1 : Outport
  wires:
  In1/1 -> Out1/1

== system GS_model/Subsystem2/Subsystem/Sensor/Magnetometer/MmModel2/Mm_ErrSet/MmErrSet/MmErrSet_Wave/MmAxisXErrSet_Wave1/Triggered Subsystem8 ==
  In1 : Inport
  Enable : EnablePort
  Out1 : Outport
  wires:
  In1/1 -> Out1/1

== system GS_model/Subsystem2/Subsystem/Sensor/Magnetometer/MmModel2/Mm_ErrSet/MmErrSet/MmErrSet_Wave/MmAxisXErrSet_Wave2/Triggered Subsystem8 ==
  In1 : Inport
  Enable : EnablePort
  Out1 : Outport
  wires:
  In1/1 -> Out1/1

== system GS_model/Subsystem2/Subsystem/Sensor/Magnetometer/MmModel2/Mm_ErrSet/MmErrSet/MmErrSet_WildValue/MmAxisXErrSet_WildValue/Triggered Subsystem8 ==
  In1 : Inport
  Enable : EnablePort
  Out1 : Outport
  wires:
  In1/1 -> Out1/1

== system GS_model/Subsystem2/Subsystem/Sensor/Magnetometer/MmModel2/Mm_ErrSet/MmErrSet/MmErrSet_WildValue/MmAxisXErrSet_WildValue1/Triggered Subsystem8 ==
  In1 : Inport
  Enable : EnablePort
  Out1 : Outport
  wires:
  In1/1 -> Out1/1

== system GS_model/Subsystem2/Subsystem/Sensor/Magnetometer/MmModel2/Mm_ErrSet/MmErrSet/MmErrSet_WildValue/MmAxisXErrSet_WildValue2/Triggered Subsystem8 ==
  In1 : Inport
  Enable : EnablePort
  Out1 : Outport
  wires:
  In1/1 -> Out1/1

== system GS_model/Subsystem2/Subsystem/Sensor/Magnetometer/MmModel3/Mm_ErrSet/MmErrSet/MmErrSet_Constant/MmAxisXErrSet_Constant/Triggered Subsystem8 ==
  In1 : Inport
  Enable : EnablePort
  Out1 : Outport
  wires:
  In1/1 -> Out1/1

== system GS_model/Subsystem2/Subsystem/Sensor/Magnetometer/MmModel3/Mm_ErrSet/MmErrSet/MmErrSet_Constant/MmAxisXErrSet_Constant1/Triggered Subsystem8 ==
  In1 : Inport
  Enable : EnablePort
  Out1 : Outport
  wires:
  In1/1 -> Out1/1

== system GS_model/Subsystem2/Subsystem/Sensor/Magnetometer/MmModel3/Mm_ErrSet/MmErrSet/MmErrSet_Constant/MmAxisXErrSet_Constant2/Triggered Subsystem8 ==
  In1 : Inport
  Enable : EnablePort
  Out1 : Outport
  wires:
  In1/1 -> Out1/1

== system GS_model/Subsystem2/Subsystem/Sensor/Magnetometer/MmModel3/Mm_ErrSet/MmErrSet/MmErrSet_Jump/MmAxisXErrSet_Jump/Triggered Subsystem8 ==
  In1 : Inport
  Enable : EnablePort
  Out1 : Outport
  wires:
  In1/1 -> Out1/1

== system GS_model/Subsystem2/Subsystem/Sensor/Magnetometer/MmModel3/Mm_ErrSet/MmErrSet/MmErrSet_Jump/MmAxisXErrSet_Jump1/Triggered Subsystem8 ==
  In1 : Inport
  Enable : EnablePort
  Out1 : Outport
  wires:
  In1/1 -> Out1/1

== system GS_model/Subsystem2/Subsystem/Sensor/Magnetometer/MmModel3/Mm_ErrSet/MmErrSet/MmErrSet_Jump/MmAxisXErrSet_Jump2/Triggered Subsystem8 ==
  In1 : Inport
  Enable : EnablePort
  Out1 : Outport
  wires:
  In1/1 -> Out1/1

== system GS_model/Subsystem2/Subsystem/Sensor/Magnetometer/MmModel3/Mm_ErrSet/MmErrSet/MmErrSet_Wave/MmAxisXErrSet_Wave/Triggered Subsystem8 ==
  In1 : Inport
  Enable : EnablePort
  Out1 : Outport
  wires:
  In1/1 -> Out1/1

== system GS_model/Subsystem2/Subsystem/Sensor/Magnetometer/MmModel3/Mm_ErrSet/MmErrSet/MmErrSet_Wave/MmAxisXErrSet_Wave1/Triggered Subsystem8 ==
  In1 : Inport
  Enable : EnablePort
  Out1 : Outport
  wires:
  In1/1 -> Out1/1

== system GS_model/Subsystem2/Subsystem/Sensor/Magnetometer/MmModel3/Mm_ErrSet/MmErrSet/MmErrSet_Wave/MmAxisXErrSet_Wave2/Triggered Subsystem8 ==
  In1 : Inport
  Enable : EnablePort
  Out1 : Outport
  wires:
  In1/1 -> Out1/1

== system GS_model/Subsystem2/Subsystem/Sensor/Magnetometer/MmModel3/Mm_ErrSet/MmErrSet/MmErrSet_WildValue/MmAxisXErrSet_WildValue/Triggered Subsystem8 ==
  In1 : Inport
  Enable : EnablePort
  Out1 : Outport
  wires:
  In1/1 -> Out1/1

== system GS_model/Subsystem2/Subsystem/Sensor/Magnetometer/MmModel3/Mm_ErrSet/MmErrSet/MmErrSet_WildValue/MmAxisXErrSet_WildValue1/Triggered Subsystem8 ==
  In1 : Inport
  Enable : EnablePort
  Out1 : Outport
  wires:
  In1/1 -> Out1/1

== system GS_model/Subsystem2/Subsystem/Sensor/Magnetometer/MmModel3/Mm_ErrSet/MmErrSet/MmErrSet_WildValue/MmAxisXErrSet_WildValue2/Triggered Subsystem8 ==
  In1 : Inport
  Enable : EnablePort
  Out1 : Outport
  wires:
  In1/1 -> Out1/1

== system GS_model/Subsystem2/Subsystem/Sensor/Magnetometer/MmModel4/Mm_ErrSet/MmErrSet/MmErrSet_Constant/MmAxisXErrSet_Constant/Triggered Subsystem8 ==
  In1 : Inport
  Enable : EnablePort
  Out1 : Outport
  wires:
  In1/1 -> Out1/1

== system GS_model/Subsystem2/Subsystem/Sensor/Magnetometer/MmModel4/Mm_ErrSet/MmErrSet/MmErrSet_Constant/MmAxisXErrSet_Constant1/Triggered Subsystem8 ==
  In1 : Inport
  Enable : EnablePort
  Out1 : Outport
  wires:
  In1/1 -> Out1/1

== system GS_model/Subsystem2/Subsystem/Sensor/Magnetometer/MmModel4/Mm_ErrSet/MmErrSet/MmErrSet_Constant/MmAxisXErrSet_Constant2/Triggered Subsystem8 ==
  In1 : Inport
  Enable : EnablePort
  Out1 : Outport
  wires:
  In1/1 -> Out1/1

== system GS_model/Subsystem2/Subsystem/Sensor/Magnetometer/MmModel4/Mm_ErrSet/MmErrSet/MmErrSet_Jump/MmAxisXErrSet_Jump/Triggered Subsystem8 ==
  In1 : Inport
  Enable : EnablePort
  Out1 : Outport
  wires:
  In1/1 -> Out1/1

== system GS_model/Subsystem2/Subsystem/Sensor/Magnetometer/MmModel4/Mm_ErrSet/MmErrSet/MmErrSet_Jump/MmAxisXErrSet_Jump1/Triggered Subsystem8 ==
  In1 : Inport
  Enable : EnablePort
  Out1 : Outport
  wires:
  In1/1 -> Out1/1

== system GS_model/Subsystem2/Subsystem/Sensor/Magnetometer/MmModel4/Mm_ErrSet/MmErrSet/MmErrSet_Jump/MmAxisXErrSet_Jump2/Triggered Subsystem8 ==
  In1 : Inport
  Enable : EnablePort
  Out1 : Outport
  wires:
  In1/1 -> Out1/1

== system GS_model/Subsystem2/Subsystem/Sensor/Magnetometer/MmModel4/Mm_ErrSet/MmErrSet/MmErrSet_Wave/MmAxisXErrSet_Wave/Triggered Subsystem8 ==
  In1 : Inport
  Enable : EnablePort
  Out1 : Outport
  wires:
  In1/1 -> Out1/1

== system GS_model/Subsystem2/Subsystem/Sensor/Magnetometer/MmModel4/Mm_ErrSet/MmErrSet/MmErrSet_Wave/MmAxisXErrSet_Wave1/Triggered Subsystem8 ==
  In1 : Inport
  Enable : EnablePort
  Out1 : Outport
  wires:
  In1/1 -> Out1/1

== system GS_model/Subsystem2/Subsystem/Sensor/Magnetometer/MmModel4/Mm_ErrSet/MmErrSet/MmErrSet_Wave/MmAxisXErrSet_Wave2/Triggered Subsystem8 ==
  In1 : Inport
  Enable : EnablePort
  Out1 : Outport
  wires:
  In1/1 -> Out1/1

== system GS_model/Subsystem2/Subsystem/Sensor/Magnetometer/MmModel4/Mm_ErrSet/MmErrSet/MmErrSet_WildValue/MmAxisXErrSet_WildValue/Triggered Subsystem8 ==
  In1 : Inport
  Enable : EnablePort
  Out1 : Outport
  wires:
  In1/1 -> Out1/1

== system GS_model/Subsystem2/Subsystem/Sensor/Magnetometer/MmModel4/Mm_ErrSet/MmErrSet/MmErrSet_WildValue/MmAxisXErrSet_WildValue1/Triggered Subsystem8 ==
  In1 : Inport
  Enable : EnablePort
  Out1 : Outport
  wires:
  In1/1 -> Out1/1

== system GS_model/Subsystem2/Subsystem/Sensor/Magnetometer/MmModel4/Mm_ErrSet/MmErrSet/MmErrSet_WildValue/MmAxisXErrSet_WildValue2/Triggered Subsystem8 ==
  In1 : Inport
  Enable : EnablePort
  Out1 : Outport
  wires:
  In1/1 -> Out1/1

== system GS_model/Subsystem2/Subsystem/PhysicsModel/Environment/Sun  press torque/Sun  press torque2/Sun  press torque/+Y SunPanel/Compute press of sun radiation/1//r/If Action Subsystem1 ==
  In1 : Inport
  Action Port : ActionPort  ActionType=else
  Fcn : Fcn  Expr=1/sqrt(u)
  Out1 : Outport
  wires:
  Fcn/1 -> Out1/1
  In1/1 -> Fcn/1

== system GS_model/Subsystem2/Subsystem/PhysicsModel/Environment/Sun  press torque/Sun  press torque2/Sun  press torque/+Y SunPanel/Compute press of sun radiation/1//r/If Action Subsystem2 ==
  Action Port : ActionPort  ActionType=then
  Constant : Constant  Value=0
  Out1 : Outport  InitialOutput=0
  wires:
  Constant/1 -> Out1/1

== system GS_model/Subsystem2/Subsystem/PhysicsModel/Environment/Sun  press torque/Sun  press torque2/Sun  press torque/-Y SunPanel/Compute press of sun radiation/1//r/If Action Subsystem1 ==
  In1 : Inport
  Action Port : ActionPort  ActionType=else
  Fcn : Fcn  Expr=1/sqrt(u)
  Out1 : Outport
  wires:
  In1/1 -> Fcn/1
  Fcn/1 -> Out1/1

== system GS_model/Subsystem2/Subsystem/PhysicsModel/Environment/Sun  press torque/Sun  press torque2/Sun  press torque/-Y SunPanel/Compute press of sun radiation/1//r/If Action Subsystem2 ==
  Action Port : ActionPort  ActionType=then
  Constant : Constant  Value=0
  Out1 : Outport  InitialOutput=0
  wires:
  Constant/1 -> Out1/1

== system GS_model/Subsystem2/Subsystem/PhysicsModel/Environment/Sun  press torque/Sun  press torque2/Sun  press torque/Torque from   satalite board/Torque from  board perpendicular to z axis /Compute press of sun radiation/1//r ==
  In1 : Inport
  Constant : Constant  Value=0
  If : If  IfExpression=u1== 0
  If Action Subsystem1 : Subsystem  TreatAsAtomicUnit=on
  If Action Subsystem2 : Subsystem  TreatAsAtomicUnit=on
  Merge : Merge
  Out1 : Outport
  wires:
  Constant/1 -> If Action Subsystem2/1(In1)
  If/1 -> If Action Subsystem2/Action
  If/2 -> If Action Subsystem1/Action
  If Action Subsystem1/1(Out1) -> Merge/2
  If Action Subsystem2/1(Out1) -> Merge/1
  Merge/1 -> Out1/1
  In1/1 -> If/1, If Action Subsystem1/1(In1)

== system GS_model/Subsystem2/Subsystem/PhysicsModel/Environment/Sun  press torque/Sun  press torque2/Sun  press torque/Torque from   satalite board/Torque from board perpendicular to x axis/Compute press of sun radiation/1//r ==
  In1 : Inport
  If : If  IfExpression=u1== 0
  If Action Subsystem1 : Subsystem  TreatAsAtomicUnit=on
  If Action Subsystem2 : Subsystem  TreatAsAtomicUnit=on
  Merge : Merge
  Out1 : Outport
  wires:
  If/1 -> If Action Subsystem2/Action
  If/2 -> If Action Subsystem1/Action
  If Action Subsystem1/1(Out1) -> Merge/2
  If Action Subsystem2/1(Out1) -> Merge/1
  Merge/1 -> Out1/1
  In1/1 -> If/1, If Action Subsystem1/1(In1)

== system GS_model/Subsystem2/Subsystem/PhysicsModel/Environment/Sun  press torque/Sun  press torque2/Sun  press torque/Torque from   satalite board/Torque from board perpendicular to y axis/Compute press of sun radiation1/1//r ==
  In1 : Inport
  If : If  IfExpression=u1== 0
  If Action Subsystem1 : Subsystem  TreatAsAtomicUnit=on
  If Action Subsystem2 : Subsystem  TreatAsAtomicUnit=on
  Merge : Merge
  Out1 : Outport
  wires:
  If/1 -> If Action Subsystem2/Action
  If/2 -> If Action Subsystem1/Action
  If Action Subsystem1/1(Out1) -> Merge/2
  If Action Subsystem2/1(Out1) -> Merge/1
  Merge/1 -> Out1/1
  In1/1 -> If/1, If Action Subsystem1/1(In1)

== system GS_model/Subsystem2/Subsystem/PhysicsModel/Environment/Sun  press torque/Sun  press torque2/Sun  press torque/Torque from   satalite board/Torque from  board perpendicular to z axis /Compute press of sun radiation/1//r/If Action Subsystem1 ==
  In1 : Inport
  Action Port : ActionPort  ActionType=else
  Fcn : Fcn  Expr=1/sqrt(u)
  Out1 : Outport
  wires:
  In1/1 -> Fcn/1
  Fcn/1 -> Out1/1

== system GS_model/Subsystem2/Subsystem/PhysicsModel/Environment/Sun  press torque/Sun  press torque2/Sun  press torque/Torque from   satalite board/Torque from  board perpendicular to z axis /Compute press of sun radiation/1//r/If Action Subsystem2 ==
  In1 : Inport
  Action Port : ActionPort  ActionType=then
  Out1 : Outport  InitialOutput=0
  wires:
  In1/1 -> Out1/1

== system GS_model/Subsystem2/Subsystem/PhysicsModel/Environment/Sun  press torque/Sun  press torque2/Sun  press torque/Torque from   satalite board/Torque from board perpendicular to x axis/Compute press of sun radiation/1//r/If Action Subsystem1 ==
  In1 : Inport
  Action Port : ActionPort  ActionType=else
  Fcn : Fcn  Expr=1/sqrt(u)
  Out1 : Outport
  wires:
  In1/1 -> Fcn/1
  Fcn/1 -> Out1/1

== system GS_model/Subsystem2/Subsystem/PhysicsModel/Environment/Sun  press torque/Sun  press torque2/Sun  press torque/Torque from   satalite board/Torque from board perpendicular to x axis/Compute press of sun radiation/1//r/If Action Subsystem2 ==
  Action Port : ActionPort  ActionType=then
  Constant : Constant  Value=0
  Out1 : Outport  InitialOutput=0
  wires:
  Constant/1 -> Out1/1

== system GS_model/Subsystem2/Subsystem/PhysicsModel/Environment/Sun  press torque/Sun  press torque2/Sun  press torque/Torque from   satalite board/Torque from board perpendicular to y axis/Compute press of sun radiation1/1//r/If Action Subsystem1 ==
  In1 : Inport
  Action Port : ActionPort  ActionType=else
  Fcn : Fcn  Expr=1/sqrt(u)
  Out1 : Outport
  wires:
  In1/1 -> Fcn/1
  Fcn/1 -> Out1/1

== system GS_model/Subsystem2/Subsystem/PhysicsModel/Environment/Sun  press torque/Sun  press torque2/Sun  press torque/Torque from   satalite board/Torque from board perpendicular to y axis/Compute press of sun radiation1/1//r/If Action Subsystem2 ==
  Action Port : ActionPort  ActionType=then
  Constant : Constant  Value=0
  Out1 : Outport  InitialOutput=0
  wires:
  Constant/1 -> Out1/1

== matlab function GS_model/Subsystem2/Subsystem/PhysicsModel/Orbit/MATLAB Function ==
  data: R_84 input; L_Geodetic output; B_Geodetic output; H_Geodetic output; L_Geocentric output; B_Geocentric output; H_Geocentric output
function [L_Geodetic, B_Geodetic, H_Geodetic, L_Geocentric, B_Geocentric,H_Geocentric] = RV2LBH(R_84)
% 根据84系下的卫星位置矢量计算经纬高
X = R_84(1);
Y = R_84(2);
Z = R_84(3);
% X=4514.634013358707e3;     Y=0.000000;    Z=4490.458200885586e3;
% X=3909739.603015826084;   Y= 2257289.2122553256;    Z=4490402.537094932050;
% X=-341629.666030938911717;    Y=-5735804.583868882618845;    Z=3780561.440661161206663;
a = 6378137;
b = 6356752;
e2 = (a^2-b^2)/a^2;
ep2 = (a^2-b^2)/b^2;
theta = atan(Z*a/sqrt(X^2+Y^2)/b);

L_Geodetic = atan2(Y,X);
B_Geodetic = atan((Z+ep2*b*(sin(theta))^3)/(sqrt(X^2+Y^2)-e2*a*(cos(theta))^3));

N = a/sqrt(1-e2*sin(B_Geodetic)^2);
H_Geodetic = sqrt(X^2+Y^2)/cos(B_Geodetic)-N;

L_Geocentric = L_Geodetic;
B_Geocentric = atan(Z/sqrt(X^2+Y^2));
H_Geocentric = sqrt(X^2+Y^2+Z^2);

== matlab function GS_model/Subsystem2/Subsystem/PhysicsModel/Environment1/MATLAB Function ==
  data: JDC_2000 input; R_Sun output; AscDec_Sun output
function [R_Sun, AscDec_Sun] = SunParamCal(JDC_2000)
% persistent tick;
% if isempty(tick)
%     tick = 0;
% end
% tick = tick+1;
% disp(tick)
% 计算太阳在惯性系下的位置矢量及赤经赤纬
M = 357.5256 + 35999.049*JDC_2000;
lamM = 282.94 + M + 1.9144*sind(M) + 0.02*sind(2 * M);
rs = (149.619 - 2.499*cosd(M) - 0.021*cosd(2 * M))*1e9;
m33 = Rx(-23.43929111*pi/180);
v31 = [rs*cosd(lamM); rs*sind(lamM);0.0];%[cosd(lamM); sind(lamM);0.0];%
R_Sun = m33*v31;
AscDec_Sun = [0;0];
AscDec_Sun(1) = atan2(R_Sun(2),R_Sun(1));
AscDec_Sun(2) = atan2(R_Sun(3),sqrt(R_Sun(1)^2+R_Sun(2)^2));
% y =[R_Sun;Asc_Sun;Dec_Sun];
end
function A = Rx(alpha)
A = [1 0 0;0 cos(alpha) sin(alpha);0 -sin(alpha) cos(alpha)];
end

== matlab function GS_model/Subsystem2/Subsystem/PhysicsModel/Orbit/MATLAB Function1 ==
  data: RV_i output; Orbit input
function RV_i = Orbit2RV(Orbit)
% 瞬根轨道转惯性系RV
a = Orbit(1);
e = Orbit(2);
i = Orbit(3);
OMG = Orbit(4);
omg = Orbit(5);
f = Orbit(6);
p=a*(1-e^2);
r0=p/(1+e*cos(f));
miu = 3.9860044e14;
% v0=sqrt(mu*(2/r0-1/a));
% sg=e*sin(f)/sqrt(1+e^2+2*e*cos(f));
% cg=sqrt(1-sg^2);
x0=r0*(cos(omg+f)*cos(OMG)-sin(omg+f)*cos(i)*sin(OMG));
y0=r0*(cos(omg+f)*sin(OMG)+sin(omg+f)*cos(i)*cos(OMG));
z0=r0*sin(omg+f)*sin(i);
R_i = [x0;y0;z0];
% x0=1184844.6264962;y0=-3166067.5090052;z0=6192267.2136932;
% vx0=v0*(sg*(cos(omg+f)*cos(OMG)-sin(omg+f)*cos(i)*sin(OMG))+cg*(-sin(omg+f)*cos(OMG)-cos(omg+f)*cos(i)*sin(OMG)));% x肖业伦P53
% vy0=v0*(sg*(cos(omg+f)*sin(OMG)+sin(omg+f)*cos(i)*cos(OMG))+cg*(-sin(omg+f)*sin(OMG)+cos(omg+f)*cos(i)*cos(OMG)));
% vz0=v0*(sg*sin(omg+f)*sin(i)+cg*cos(omg+f)*sin(i));
sp=[cos(omg)*cos(OMG)-sin(omg)*sin(OMG)*cos(i);cos(omg)*sin(OMG)+sin(omg)*cos(OMG)*cos(i);sin(omg)*sin(i)];
sq=[-sin(omg)*cos(OMG)-cos(omg)*sin(OMG)*cos(i);-sin(omg)*sin(OMG)+cos(omg)*cos(OMG)*cos(i);cos(omg)*sin(i)];
vx0=sqrt(miu/a/(1-e^2))*(-sin(f)*sp(1)+(e+cos(f))*sq(1));
vy0=sqrt(miu/a/(1-e^2))*(-sin(f)*sp(2)+(e+cos(f))*sq(2));
vz0=sqrt(miu/a/(1-e^2))*(-sin(f)*sp(3)+(e+cos(f))*sq(3));
V_i = [vx0;vy0;vz0];
RV_i=[R_i;V_i];
